simulink model "CircuitWithStates"  (R2012b)
settings: Solver=ode45  StartTime=0.0  StopTime=10.0  RelTol=1e-3
settings Model: Creator=sz609516  LastModifiedBy=sz609516
settings DataIOCC: SignalLoggingSaveFormat=ModelDataLogs
settings DebuggingCC: FcnCallInpInsideContextMsg=EnableAllAsWarning
settings GRTTargetCC: CombineOutputUpdateFcns=off  GRTInterface=on

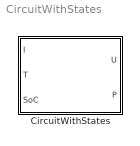
== system CircuitWithStates ==
  CircuitWithStates : Subsystem

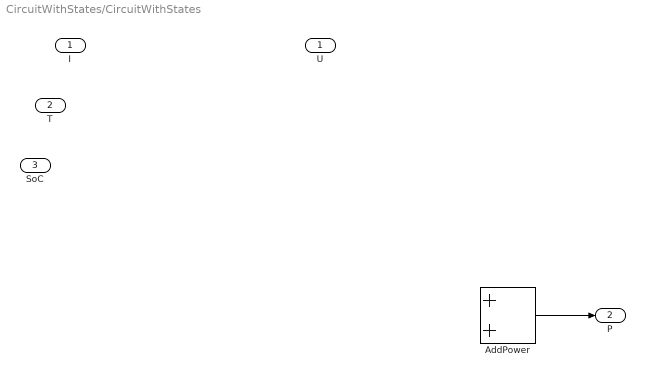
== system CircuitWithStates/CircuitWithStates ==
  I : Inport
  T : Inport  Port=2
  SoC : Inport  Port=3
  AddPower : Sum
  U : Outport
  P : Outport  Port=2
  wires:
  AddPower/1 -> P/1
